simulink model "HybridSystem_Plant_Joystick"  (R2017a)
settings: Solver=ode3  StartTime=0.0  StopTime=500  FixedStep=0.01  RelTol=1e-3  EnableMultiTasking=on
StartFcn:
  | clear;clc;close all;
libraries: simulink x4, aerolibanimutils x2
settings Model: Creator=GeoLee  LastModifiedBy=gmh_n
settings DataIOCC: LimitDataPoints=on  SaveFormat=Array
settings OptimizationCC: LifeSpan=inf
settings DebuggingCC: SFUnexpectedBacktrackingDiag=warning  SFNoUnconditionalDefaultTransitionDiag=warning  SFExecutionAtInitializationDiag=none
settings HardwareCC: ProdBitPerPointer=32  ProdBitPerSizeT=32  ProdBitPerPtrDiffT=32  ProdLargestAtomicFloat=None  ProdIntDivRoundTo=Undefined  ProdEndianess=Unspecified  ProdWordSize=32  ProdHWDeviceType=32-bit Generic
settings ModelReferenceCC: PropagateSignalLabelsOutOfModel=off
settings GRTTargetCC: TargetLangStandard=C89/C90 (ANSI)  GeneratePreprocessorConditionals=Disable all
settings ConfigComp: CovMetricSettings=dw  CovHtmlReporting=on  CovSaveCumulativeToWorkspaceVar=on  CovSaveSingleToWorkspaceVar=on  CovExternalEMLEnable=off

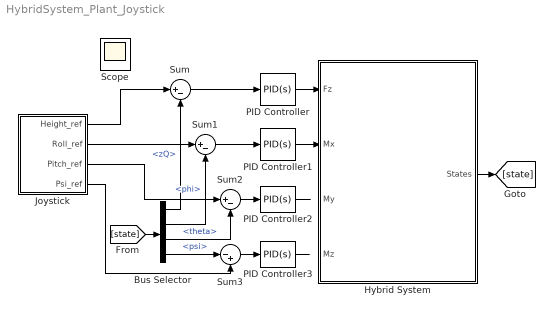
== system HybridSystem_Plant_Joystick ==
  Bus Selector : BusSelector  OutputSignals=zQ,phi,theta,psi
  Hybrid System : Subsystem
      settings: MinAlgLoopOccurrences=on
      mask Display:
      | image(imread('single_demo.png'));
      | port_label('input',1,'Fz');
      | port_label('input',2,'Mx');
      | port_label('input',3,'My');
      | port_label('input',4,'Mz');
      | 
      | port_label('output',1,'State');
  Joystick : Subsystem
  PID Controller : simulink/Continuous/PID Controller  Controller=PID  TimeDomain=Continuous-time  SampleTime=-1  IntegratorMethod=Forward Euler  FilterMethod=Forward Euler  Form=Parallel  UseFilter=on  ControllerParametersSource=internal  P=5  I=0  D=2  N=100  InitialConditionSource=internal  InitialConditionForIntegrator=0  InitialConditionForFilter=0  ExternalReset=none  LimitOutput=off  UpperSaturationLimit=inf  LowerSaturationLimit=-inf  LinearizeAsGain=on  AntiWindupMode=none  Kb=1  TrackingMode=off  Kt=1  PParamMin=[]  PParamMax=[]  IParamMin=[]  IParamMax=[]  DParamMin=[]  DParamMax=[]  NParamMin=[]  NParamMax=[]  KbParamMin=[]  KbParamMax=[]  KtParamMin=[]  KtParamMax=[]  POutMin=[]  POutMax=[]  IOutMin=[]  IOutMax=[]  DOutMin=[]  DOutMax=[]  NOutMin=[]  NOutMax=[]  KbOutMin=[]  KbOutMax=[]  KtOutMin=[]  KtOutMax=[]  IntegratorOutMin=[]  IntegratorOutMax=[]  FilterOutMin=[]  FilterOutMax=[]  SumOutMin=[]  SumOutMax=[]  SumI1OutMin=[]  SumI1OutMax=[]  SumI2OutMin=[]  SumI2OutMax=[]  SumI3OutMin=[]  SumI3OutMax=[]  SumDOutMin=[]  SumDOutMax=[]  SaturationOutMin=[]  SaturationOutMax=[]  IntegratorContinuousStateAttributes=''  IntegratorStateMustResolveToSignalObject=off  IntegratorRTWStateStorageClass=Auto  FilterContinuousStateAttributes=''  FilterStateMustResolveToSignalObject=off  FilterRTWStateStorageClass=Auto  DifferentiatorICPrevScaledInput=0  DifferentiatorOutMin=[]  DifferentiatorOutMax=[]  InitialConditionSetting=State (most efficient)
  PID Controller1 : simulink/Continuous/PID Controller  Controller=PID  TimeDomain=Continuous-time  SampleTime=-1  IntegratorMethod=Forward Euler  FilterMethod=Forward Euler  Form=Parallel  UseFilter=on  ControllerParametersSource=internal  P=0.5  I=0  D=0.2  N=100  InitialConditionSource=internal  InitialConditionForIntegrator=0  InitialConditionForFilter=0  ExternalReset=none  LimitOutput=off  UpperSaturationLimit=inf  LowerSaturationLimit=-inf  LinearizeAsGain=on  AntiWindupMode=none  Kb=1  TrackingMode=off  Kt=1  PParamMin=[]  PParamMax=[]  IParamMin=[]  IParamMax=[]  DParamMin=[]  DParamMax=[]  NParamMin=[]  NParamMax=[]  KbParamMin=[]  KbParamMax=[]  KtParamMin=[]  KtParamMax=[]  POutMin=[]  POutMax=[]  IOutMin=[]  IOutMax=[]  DOutMin=[]  DOutMax=[]  NOutMin=[]  NOutMax=[]  KbOutMin=[]  KbOutMax=[]  KtOutMin=[]  KtOutMax=[]  IntegratorOutMin=[]  IntegratorOutMax=[]  FilterOutMin=[]  FilterOutMax=[]  SumOutMin=[]  SumOutMax=[]  SumI1OutMin=[]  SumI1OutMax=[]  SumI2OutMin=[]  SumI2OutMax=[]  SumI3OutMin=[]  SumI3OutMax=[]  SumDOutMin=[]  SumDOutMax=[]  SaturationOutMin=[]  SaturationOutMax=[]  IntegratorContinuousStateAttributes=''  IntegratorStateMustResolveToSignalObject=off  IntegratorRTWStateStorageClass=Auto  FilterContinuousStateAttributes=''  FilterStateMustResolveToSignalObject=off  FilterRTWStateStorageClass=Auto  DifferentiatorICPrevScaledInput=0  DifferentiatorOutMin=[]  DifferentiatorOutMax=[]  InitialConditionSetting=State (most efficient)
  PID Controller2 : simulink/Continuous/PID Controller  Controller=PID  TimeDomain=Continuous-time  SampleTime=-1  IntegratorMethod=Forward Euler  FilterMethod=Forward Euler  Form=Parallel  UseFilter=on  ControllerParametersSource=internal  P=0.5  I=0  D=0.2  N=100  InitialConditionSource=internal  InitialConditionForIntegrator=0  InitialConditionForFilter=0  ExternalReset=none  LimitOutput=off  UpperSaturationLimit=inf  LowerSaturationLimit=-inf  LinearizeAsGain=on  AntiWindupMode=none  Kb=1  TrackingMode=off  Kt=1  PParamMin=[]  PParamMax=[]  IParamMin=[]  IParamMax=[]  DParamMin=[]  DParamMax=[]  NParamMin=[]  NParamMax=[]  KbParamMin=[]  KbParamMax=[]  KtParamMin=[]  KtParamMax=[]  POutMin=[]  POutMax=[]  IOutMin=[]  IOutMax=[]  DOutMin=[]  DOutMax=[]  NOutMin=[]  NOutMax=[]  KbOutMin=[]  KbOutMax=[]  KtOutMin=[]  KtOutMax=[]  IntegratorOutMin=[]  IntegratorOutMax=[]  FilterOutMin=[]  FilterOutMax=[]  SumOutMin=[]  SumOutMax=[]  SumI1OutMin=[]  SumI1OutMax=[]  SumI2OutMin=[]  SumI2OutMax=[]  SumI3OutMin=[]  SumI3OutMax=[]  SumDOutMin=[]  SumDOutMax=[]  SaturationOutMin=[]  SaturationOutMax=[]  IntegratorContinuousStateAttributes=''  IntegratorStateMustResolveToSignalObject=off  IntegratorRTWStateStorageClass=Auto  FilterContinuousStateAttributes=''  FilterStateMustResolveToSignalObject=off  FilterRTWStateStorageClass=Auto  DifferentiatorICPrevScaledInput=0  DifferentiatorOutMin=[]  DifferentiatorOutMax=[]  InitialConditionSetting=State (most efficient)
  PID Controller3 : simulink/Continuous/PID Controller  Controller=PID  TimeDomain=Continuous-time  SampleTime=-1  IntegratorMethod=Forward Euler  FilterMethod=Forward Euler  Form=Parallel  UseFilter=on  ControllerParametersSource=internal  P=0.5  I=0  D=0.2  N=100  InitialConditionSource=internal  InitialConditionForIntegrator=0  InitialConditionForFilter=0  ExternalReset=none  LimitOutput=off  UpperSaturationLimit=inf  LowerSaturationLimit=-inf  LinearizeAsGain=on  AntiWindupMode=none  Kb=1  TrackingMode=off  Kt=1  PParamMin=[]  PParamMax=[]  IParamMin=[]  IParamMax=[]  DParamMin=[]  DParamMax=[]  NParamMin=[]  NParamMax=[]  KbParamMin=[]  KbParamMax=[]  KtParamMin=[]  KtParamMax=[]  POutMin=[]  POutMax=[]  IOutMin=[]  IOutMax=[]  DOutMin=[]  DOutMax=[]  NOutMin=[]  NOutMax=[]  KbOutMin=[]  KbOutMax=[]  KtOutMin=[]  KtOutMax=[]  IntegratorOutMin=[]  IntegratorOutMax=[]  FilterOutMin=[]  FilterOutMax=[]  SumOutMin=[]  SumOutMax=[]  SumI1OutMin=[]  SumI1OutMax=[]  SumI2OutMin=[]  SumI2OutMax=[]  SumI3OutMin=[]  SumI3OutMax=[]  SumDOutMin=[]  SumDOutMax=[]  SaturationOutMin=[]  SaturationOutMax=[]  IntegratorContinuousStateAttributes=''  IntegratorStateMustResolveToSignalObject=off  IntegratorRTWStateStorageClass=Auto  FilterContinuousStateAttributes=''  FilterStateMustResolveToSignalObject=off  FilterRTWStateStorageClass=Auto  DifferentiatorICPrevScaledInput=0  DifferentiatorOutMin=[]  DifferentiatorOutMax=[]  InitialConditionSetting=State (most efficient)
  Sum : Sum  Inputs=|+-
  Sum1 : Sum  Inputs=|+-
  Sum2 : Sum  Inputs=|+-
  Sum3 : Sum  Inputs=|-+
  Scope : Scope
  wires:
  Hybrid System/1(States) -> [state]
  [state] -> Bus Selector/1
  Bus Selector/1 -> Sum/2  "<zQ>"
  Sum/1 -> PID Controller/1
  PID Controller/1 -> Hybrid System/1(Fz)
  Joystick/1(Height_ref) -> Sum/1
  PID Controller1/1 -> Hybrid System/2(Mx)
  Sum1/1 -> PID Controller1/1
  Joystick/2(Roll_ref) -> Sum1/1
  Bus Selector/2 -> Sum1/2  "<phi>"
  PID Controller2/1 -> ?
  Sum2/1 -> PID Controller2/1
  Bus Selector/3 -> Sum2/2  "<theta>"
  PID Controller3/1 -> ?
  Sum3/1 -> PID Controller3/1
  Bus Selector/4 -> Sum3/1  "<psi>"
  Joystick/3(Pitch_ref) -> Sum2/1
  Joystick/4(Psi_ref) -> Sum3/2

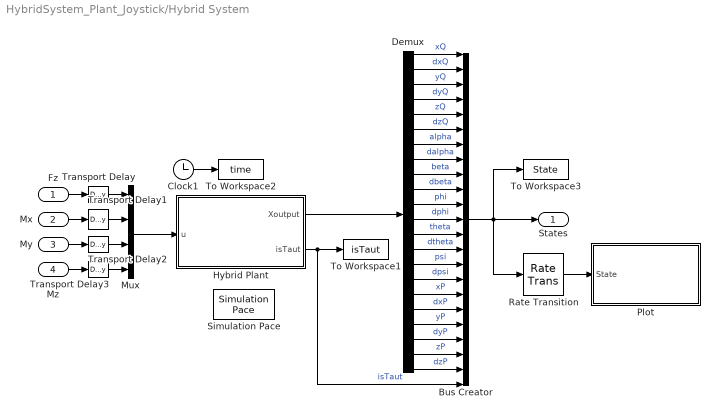
== system HybridSystem_Plant_Joystick/Hybrid System ==
  Fz : Inport
  Mx : Inport  Port=2
  My : Inport  Port=3
  Mz : Inport  Port=4
  Bus Creator : BusCreator  Inputs=23
  Clock1 : Clock
  Demux : Demux  Outputs=22
  Hybrid Plant : Stateflow chart  TreatAsAtomicUnit=on
      settings: MinAlgLoopOccurrences=on
  Mux : Mux
  Plot : Stateflow chart  TreatAsAtomicUnit=on
  Rate Transition : RateTransition  OutPortSampleTime=0.05
  Simulation Pace : aerolibanimutils/Simulation Pace  SimulationPace=1  SleepMode=MATLAB Thread  OutputPaceError=off  SampleTime=-1
  To Workspace1 : ToWorkspace  VariableName=isTaut  SampleTime=-1
  To Workspace2 : ToWorkspace  VariableName=time  SampleTime=-1
  To Workspace3 : ToWorkspace  VariableName=State  SampleTime=-1
  Transport Delay{,1..3} (4 alike) : TransportDelay  DelayTime=0.001
  States : Outport
  wires:
  Demux/7 -> Bus Creator/7  "alpha"
  Demux/3 -> Bus Creator/3  "yQ"
  Demux/21 -> Bus Creator/21  "zP"
  Demux/2 -> Bus Creator/2  "dxQ"
  Demux/22 -> Bus Creator/22  "dzP"
  Demux/20 -> Bus Creator/20  "dyP"
  Demux/4 -> Bus Creator/4  "dyQ"
  Demux/8 -> Bus Creator/8  "dalpha"
  Demux/17 -> Bus Creator/17  "xP"
  Fz/1 -> Transport Delay/1
  Demux/16 -> Bus Creator/16  "dpsi"
  Demux/12 -> Bus Creator/12  "dphi"
  Demux/6 -> Bus Creator/6  "dzQ"
  Demux/18 -> Bus Creator/18  "dxP"
  Demux/5 -> Bus Creator/5  "zQ"
  Demux/9 -> Bus Creator/9  "beta"
  Demux/11 -> Bus Creator/11  "phi"
  Demux/13 -> Bus Creator/13  "theta"
  Demux/14 -> Bus Creator/14  "dtheta"
  Demux/19 -> Bus Creator/19  "yP"
  Clock1/1 -> To Workspace2/1
  Demux/15 -> Bus Creator/15  "psi"
  Demux/10 -> Bus Creator/10  "dbeta"
  Hybrid Plant/1(Xoutput) -> Demux/1
  Demux/1 -> Bus Creator/1  "xQ"
  Hybrid Plant/2(isTaut) -> Bus Creator/23, To Workspace1/1  "isTaut"
  Rate Transition/1 -> Plot/1(State)
  Bus Creator/1 -> States/1, To Workspace3/1, Rate Transition/1
  Mux/1 -> Hybrid Plant/1(u)
  Mx/1 -> Transport Delay1/1
  Mz/1 -> Transport Delay3/1
  My/1 -> Transport Delay2/1
  Transport Delay3/1 -> Mux/4
  Transport Delay2/1 -> Mux/3
  Transport Delay1/1 -> Mux/2
  Transport Delay/1 -> Mux/1

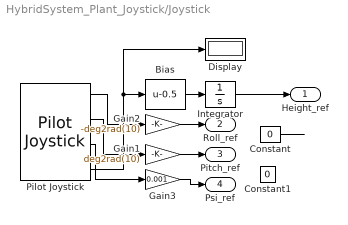
== system HybridSystem_Plant_Joystick/Joystick ==
  Bias : Bias  Bias=-0.5
  Constant : Constant  Value=0
  Constant1 : Constant  Value=0
  Display : Display
  Gain1 : Gain  Gain=deg2rad(10)
  Gain2 : Gain  Gain=-deg2rad(10)
  Gain3 : Gain  Gain=0.001
  Integrator : Integrator
  Pilot Joystick : aerolibanimutils/Pilot Joystick  JoystickID=Joystick1  OutputConfiguration=FourAxis  SampleTime=0.01
  Height_ref : Outport
  Roll_ref : Outport  Port=2
  Pitch_ref : Outport  Port=3
  Psi_ref : Outport  Port=4
  wires:
  Gain1/1 -> Pitch_ref/1
  Gain3/1 -> Psi_ref/1
  Pilot Joystick/4 -> Display/1, Bias/1
  Gain2/1 -> Roll_ref/1
  Bias/1 -> Integrator/1
  Pilot Joystick/3 -> Gain3/1
  Pilot Joystick/1 -> Gain2/1
  Pilot Joystick/2 -> Gain1/1
  Integrator/1 -> Height_ref/1
  Constant/1 -> ?

== stateflow chart HybridSystem_Plant_Joystick/Hybrid System/Plot ==
  state Plot
    entry:
    fig = ml.figure();
    phandles = ml.LG_plot_initial( fig,State);
    du:
    ml.LG_plot_update(fig,State,phandles);
  (default) -> Plot
  data: State input double size=23; fig local ml; phandles local ml

== stateflow chart HybridSystem_Plant_Joystick/Hybrid System/Hybrid Plant ==
  settings: updateMethod=CONTINUOUS  sampleTime=0.01
  state NotTaut
    % free mode
    en:
    isTaut = 0;
    Xfree = ml.LG_jump2free(X);
    du:
    Xfree_dot=ml.LG_f_free(u,Xfree);
    Xoutput = ml.LG_output_free(Xfree);
    ex:
    X=ml.LG_output_free(Xfree);
  state Taut
    % taut mode
    en:
    isTaut = 1;
    [Xtaut,X]=ml.LG_jump2taut(X);
    du:
    Xtaut_dot=ml.LG_f_taut(u,Xtaut);
    [Xoutput] = ml.LG_output_taut(Xtaut);
    ex:
    X=ml.LG_output_taut(Xtaut);
  (default) -> Taut : {X=ml.LG_initial(0,0,0,0,0);}
  Taut -> NotTaut : [ml.LG_isTension(u,ml.LG_f_taut(u,Xtaut),ml.LG_output_taut(Xtaut))<0]
  NotTaut -> Taut : [ml.LG_dis(Xfree)>0.5]
  data: u input size=4; Xoutput output size=22 =zeros(22,1); Xtaut local double size=16 =zeros(16,1); Xfree local double size=18; X local double size=22 =zeros(22,1); isTaut output double
  data Xtaut settings: updateMethod=SF_CONTINUOUS_TIME_DATA
  data Xfree settings: updateMethod=SF_CONTINUOUS_TIME_DATA
  data X settings: updateMethod=SF_CONTINUOUS_TIME_DATA
